simulink model "DC_moteor_fdi1"  (R2024b)
settings: Solver=VariableStepAuto  StartTime=0.0  StopTime=inf  RelTol=1e-3
values from neighbouring files (symbols this model uses):
  Af = 0.01    [Data__MOTOR.m]    (also in Generator_Data.m = 0.0001; Generator_Datatest.m)
  Bf = 0.0002    [Data__MOTOR.m]    (also in Generator_Data.m = 2e-05; Generator_Datatest.m)
  Cc = Cc0+6*Cc0    (= 0.7)    [Data__MOTOR.m]    (also in Generator_Datatest.m)
  Cc0 = 0.1    [Data__MOTOR.m]    (also in Generator_Datatest.m)
  CurrentFaultSwitch = 0    [Data__MOTOR.m]    (also in Generator_Data.m = 1; Generator_Datatest.m)
  Jm = 0.08    [Data__MOTOR.m]    (also in Generator_Datatest.m)
  Ke = 0.139    [Data__MOTOR.m]    (also in Generator_Datatest.m)
  Le = 0.44    [Data__MOTOR.m]    (also in Generator_Datatest.m)
  rate_noise_i = 0.02*In    (= 0.22)    [Data__MOTOR.m]    (also in Generator_Data.m = 0.02; Generator_Datatest.m)
  rate_noise_w = 0.02*Wn    (= 2.96)    [Data__MOTOR.m]    (also in Generator_Data.m = 0.002; Generator_Datatest.m)
  Re = 2.4    [Data__MOTOR.m]    (also in Generator_Datatest.m)
  ResFaultSwitch = 0    [Data__MOTOR.m]    (also in Generator_Datatest.m)
  Rm = 0.01    [Data__MOTOR.m]    (also in Generator_Datatest.m)
  StartStop = 0    [Data__MOTOR.m]    (also in Generator_Data.m; Generator_Datatest.m)
  Te = 0.1    [Data__MOTOR.m]    (also in Generator_Data.m = 1; Generator_Datatest.m)
  Ua = 48    [Data__MOTOR.m]    (also in Generator_Datatest.m)
  VelocityFaultSwitch = 0    [Data__MOTOR.m]    (also in Generator_Data.m = 1; Generator_Datatest.m)
undefined symbols (not defined in the file or in its folder): dspblkCoreblockFVToolHelper, gcbh, sigbuilder_block
libraries: SignalEditorBlockLib x2
(part 1 of 3)
settings Model: Creator=belka  LastModifiedBy=Nasser
settings DebuggingCC: SignalResolutionControl=TryResolveAll
settings RTWCC: GPUComputeCapability=3.5

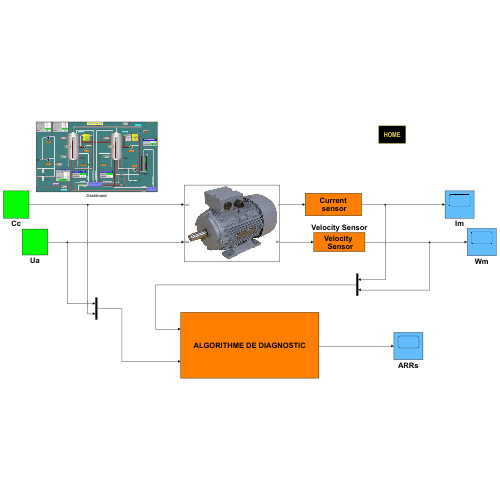
[thumbnail: Simulink's stored preview of the top-level diagram]
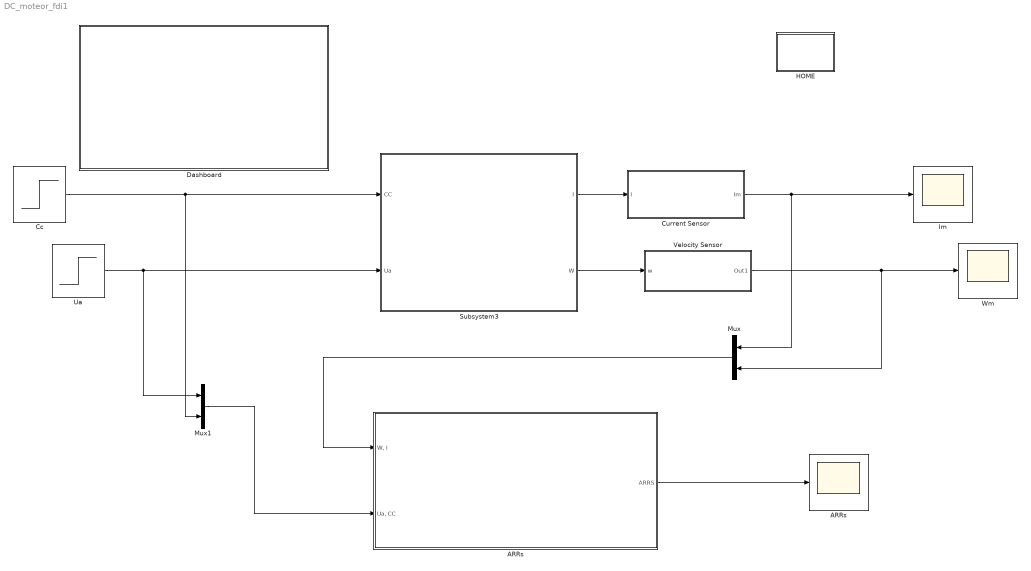
== system DC_moteor_fdi1 ==
  "  ARRs  " : Scope
  ARRs : Subsystem
      mask Display: disp('ALGORITHME DE DIAGNOSTIC')
  Cc : Step  Time=30  Before=Cc0  After=Cc  SampleTime=0
  Current Sensor : Subsystem
      mask Display: disp('Current\n sensor')
  Dashboard : Subsystem
      mask Display: image('scada.jpg');
  HOME : Subsystem
      settings: OpenFcn=MENU_SUPERVISION_MOTOR
      mask Display: disp('HOME')
  Im : Scope
  Mux : Mux  Inputs=2
  Mux1 : Mux  Inputs=2
  Subsystem3 : Subsystem
      mask Display: image('motor.jpg');
  Ua : Step  Time=0  After=Ua  SampleTime=0
  Velocity Sensor : Subsystem
      mask Display: disp('Velocity \n Sensor')
  Wm : Scope
  wires:
  Current Sensor/1(Im) -> Mux/1, Im/1
  Velocity Sensor/1(Out1) -> Mux/2, Wm/1
  Ua/1 -> Mux1/1, Subsystem3/2(Ua)
  Subsystem3/1(I) -> Current Sensor/1(I)
  Subsystem3/2(W) -> Velocity Sensor/1(w)
  Mux/1 -> ARRs/1("W, I")
  Cc/1 -> Mux1/2, Subsystem3/1(CC)
  Mux1/1 -> ARRs/2("Ua, CC")
  ARRs/1(ARRS) -> "  ARRs  "/1

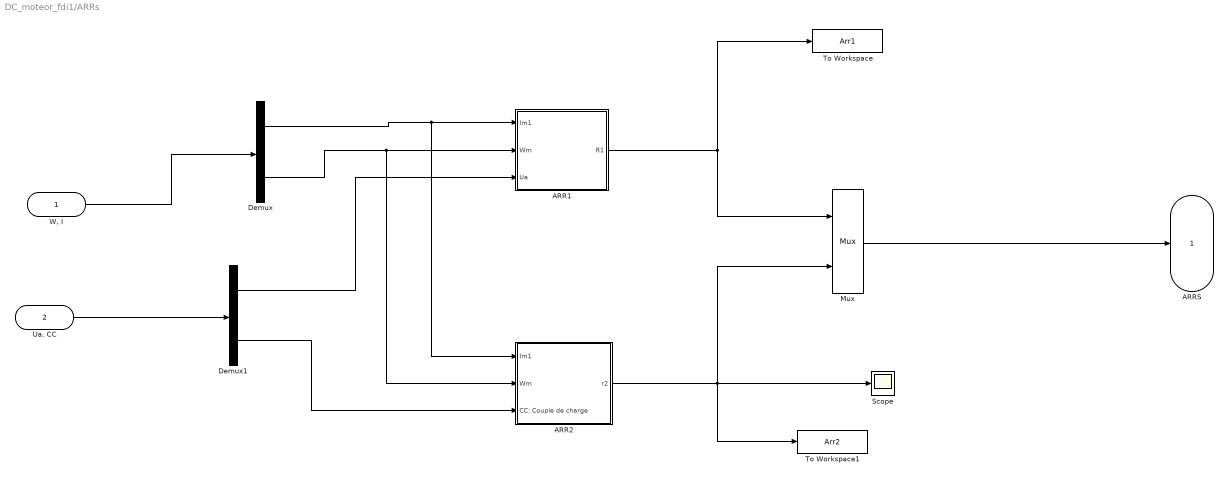
== system DC_moteor_fdi1/ARRs ==
  "W, I" : Inport
  "Ua, CC" : Inport  Port=2
  ARR1 : Subsystem
      mask Display: disp('Residu 1')
  ARR2 : Subsystem
      mask Display: disp('Residu 2')
  Demux : Demux  Outputs=2
  Demux1 : Demux  Outputs=2
  Mux : Mux  Inputs=2
  Scope : Scope
  To Workspace : ToWorkspace  VariableName=Arr1  SampleTime=Te
  To Workspace1 : ToWorkspace  VariableName=Arr2  SampleTime=Te
  ARRS : Outport  VectorParamsAs1DForOutWhenUnconnected=off
  wires:
  "W, I"/1 -> Demux/1
  Demux/1 -> ARR2/1(Im1), ARR1/1(Im1)
  Demux/2 -> ARR2/2(Wm), ARR1/2(Wm)
  "Ua, CC"/1 -> Demux1/1
  Demux1/1 -> ARR1/3(" Ua")
  Demux1/2 -> ARR2/3(CC: Couple de charge)
  ARR1/1(R1) -> To Workspace/1, Mux/1
  ARR2/1(r2) -> Scope/1, To Workspace1/1, Mux/2
  Mux/1 -> ARRS/1

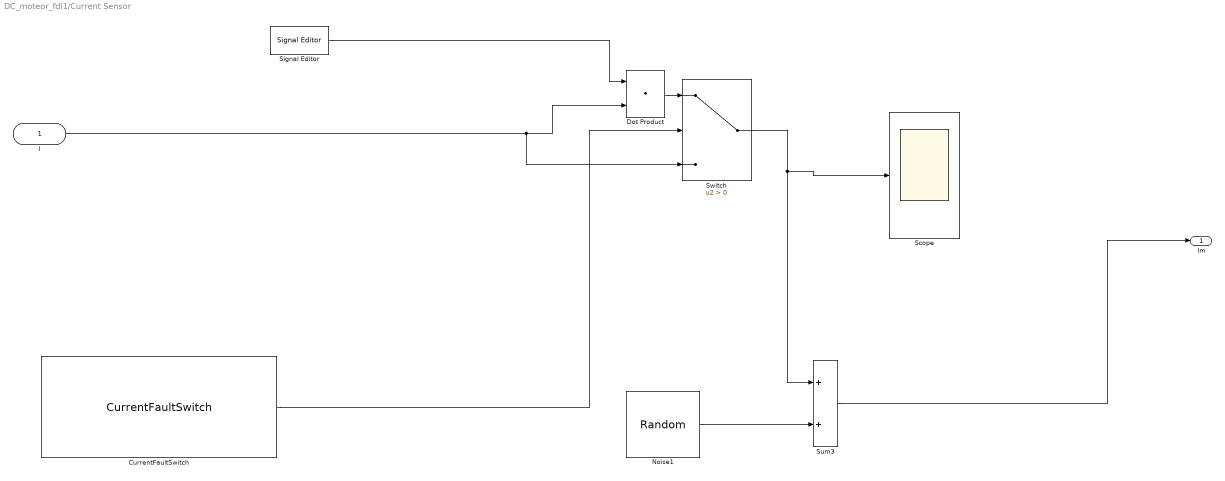
== system DC_moteor_fdi1/Current Sensor ==
  I : Inport
  CurrentFaultSwitch : Constant  Value=CurrentFaultSwitch
  Dot Product : DotProduct  OutDataTypeStr=Inherit: Inherit via internal rule
  Noise1 : UniformRandomNumber  Minimum=-rate_noise_i  Maximum=+rate_noise_i  SampleTime=0.1
  Scope : Scope
  Signal Editor : SignalEditorBlockLib/Signal Editor  FileName=CurrentFault.mat  ActiveScenario=ChuteCourant  ActiveSignal=Fault  IsBus=off  OutputBusObjectStr=Bus: BusObject  SampleTime=0  Interpolate=off  ZeroCross=off  OutputAfterFinalValue=Setting to zero  Unit=inherit  PreserveSignalName=on  ApplySigPropsToAllScenarios=on  ApplySigPropsToAllSignals=off
  Sum3 : Sum  InputSameDT=on  SaturateOnIntegerOverflow=on  OutDataTypeStr=Inherit: Same as first input
  Switch : Switch  Criteria=u2 > Threshold  SaturateOnIntegerOverflow=off  InputSameDT=off
  Im : Outport  VectorParamsAs1DForOutWhenUnconnected=off
  wires:
  Sum3/1 -> Im/1
  Noise1/1 -> Sum3/2
  Dot Product/1 -> Switch/1
  I/1 -> Switch/3, Dot Product/2
  Signal Editor/1 -> Dot Product/1
  Switch/1 -> Sum3/1, Scope/1
  CurrentFaultSwitch/1 -> Switch/2
